simulink model "TestI2C1POLLING"  (R2015b)
settings: Solver=FixedStepDiscrete  StartTime=0.0  StopTime=10.0  FixedStep=0.5  RelTol=1e-3
libraries: I2C_Lib x2, STM32_Config_Lib x1, USART_Lib x1
settings Model: Creator=Gang  LastModifiedBy=reynaudp
settings DataIOCC: SaveFormat=Array
settings OptimizationCC: OptimizeModelRefInitCode=on  LifeSpan=1
settings DebuggingCC: UnderspecifiedInitializationDetection=Classic  MergeDetectMultiDrivingBlocksExec=none  SolverPrmCheckMsg=warning
settings HardwareCC: ProdBitPerPointer=32  ProdLargestAtomicInteger=Integer  ProdWordSize=32  ProdHWDeviceType=STMicroelectronics->STM32 32-bit Cortex-M
settings RTWCC: SystemTargetFile=stm32.tlc  TemplateMakefile=stm32.tmf  Description=stm32 (Embedded Target)  GenerateReport=on  IncludeHyperlinkInReport=on  LaunchReport=on
settings CodeAppCC: IgnoreCustomStorageClasses=off  MaxIdLength=64  CustomSymbolStrType=$N$R$M  SimulinkBlockComments=off
settings STFCustomTargetCC: CodeReplacementLibrary=ARM CMSIS SIN COS  ParMdlRefBuildCompliant=on  ConcurrentExecutionCompliant=off  IncludeMdlTerminateFcn=off  GeneratePreprocessorConditionals=Use local settings  CombineOutputUpdateFcns=on  ERTCustomFileBanners=on  SupportContinuousTime=off  SupportNonInlinedSFcns=off  MATLABClassNameForMDSCustomization=Simulink.SoftwareTarget.ERTCustomization  CPPClassGenCompliant=off  GRTInterface=off  SystemTargetFile=stm32.tlc
settings ERTTargetCC: CodeReplacementLibrary=ARM CMSIS SIN COS  CompOptLevelCompliant=off  ConcurrentExecutionCompliant=off  IncludeMdlTerminateFcn=off  ERTFirstTimeCompliant=off  ModelStepFunctionPrototypeControlCompliant=off  CPPClassGenCompliant=off  UseToolchainInfoCompliant=off  ERTSrcFileBannerTemplate=sourceFileTemplate.cgt  ERTHdrFileBannerTemplate=sourceFileTemplate.cgt  ERTDataSrcFileTemplate=sourceFileTemplate.cgt  ERTDataHdrFileTemplate=sourceFileTemplate.cgt  ERTCustomFileTemplate=customRoutineProcess.tlc
settings ConfigComp: CovModelRefEnable=Off  CovSFcnEnable=off

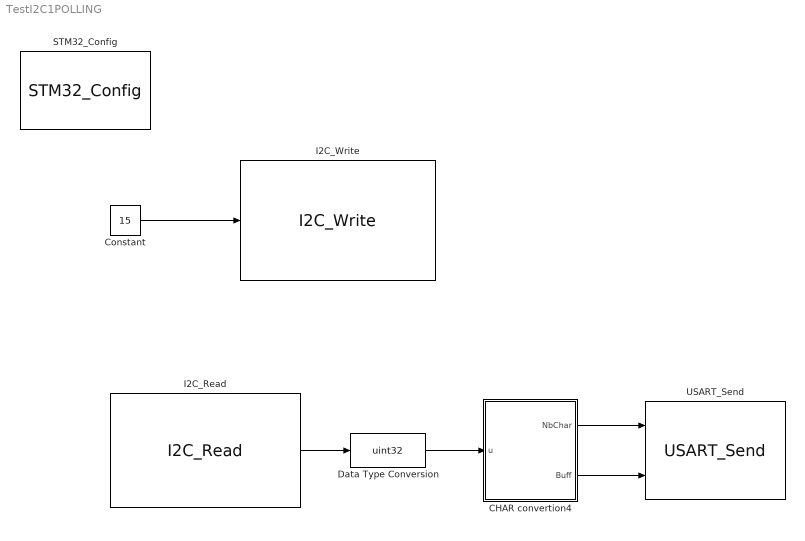
== system TestI2C1POLLING ==
  CHAR convertion4 : MATLAB Function  TreatAsAtomicUnit=on
  Constant : Constant  Value=15  OutDataTypeStr=uint8
  Data Type Conversion : DataTypeConversion  OutDataTypeStr=uint32
  I2C_Read : I2C_Lib/I2C_Read  Priority=2  i2cx=I2C1  Device_Mode=MASTER  Device_Address=62  i2c_Mode=<empty>  Target_Address=160  handler=hi2c1  Buffer_Size=2  Timeout=2000  TimeoutValue=0.001  Enable_Output=on  Error=off  CallBack=off
  I2C_Write : I2C_Lib/I2C_Write  Priority=1  i2cx=I2C1  Device_Mode=MASTER  Target_Address=160  Target_Register=1  Enable_Input=on  Data_str={18}  i2c_Mode=<empty>  Buffer_Size=1  handler=hi2c1  Timeout=50  TimeoutValue=0.001  Error=off  CallBack=off
  STM32_Config : STM32_Config_Lib/STM32_Config  Priority=0  Project_Path=.\  Config_File=TestI2C1POLLING.ioc  MCU_Name=STM32F407VGTx
  USART_Send : USART_Lib/USART_Send  USART_name=USART3  Buff_size=512  nbUsart=1  usartMode=Asynchronous  usartDma_Rx=off  usartDma_Tx=off  usartIt=on
  wires:
  I2C_Read/1 -> Data Type Conversion/1
  CHAR convertion4/1(NbChar) -> USART_Send/1
  CHAR convertion4/2(Buff) -> USART_Send/2
  Data Type Conversion/1 -> CHAR convertion4/1(u)
  Constant/1 -> I2C_Write/1

== matlab function TestI2C1POLLING/CHAR convertion4 ==
  data: NbChar output uint16 size=1; Buff output uint32 size=1; u input
function [NbChar, Buff] = convert(u)
if coder.target('Sfun')
% Executing in MATLAB, Buff is null
Buff = uint32(0);
NbChar = uint16(0);
else
% Executing in the generated code. 
buffer0 = zeros(1,20,'uint8');
strLen = int32(0);
strLen = coder.ceval('sprintf',coder.wref(buffer0),['  Byte1: 0x%02x',0], u(1));
%buffer1 = zeros(1,20,'uint8');
%strLen = coder.ceval('sprintf',coder.wref(buffer1),['  Byte1: 0x%02x\n',0], u(2));
% y = [buffer0(1:20), buffer1(1:20), 13, 10, 0];
y = [buffer0(1:20), 13, 10, 0];
Buff = coder.ceval('getBuffPtr',coder.ref(y));
NbChar = uint16(size(y,2));
end
end
%Buff = uint32(y);
%%Buff = [buffer(1:4), tmp, 13, 10, 0];
